simulink model "filter1"  (R2020b)
settings: Solver=VariableStepAuto  StartTime=0.0  StopTime=10.0  MaxStep=0.8  RelTol=1e-3
settings Model: Creator=Ravi  LastModifiedBy=Ravi
settings DataIOCC: SaveOutput=off  SaveTime=off

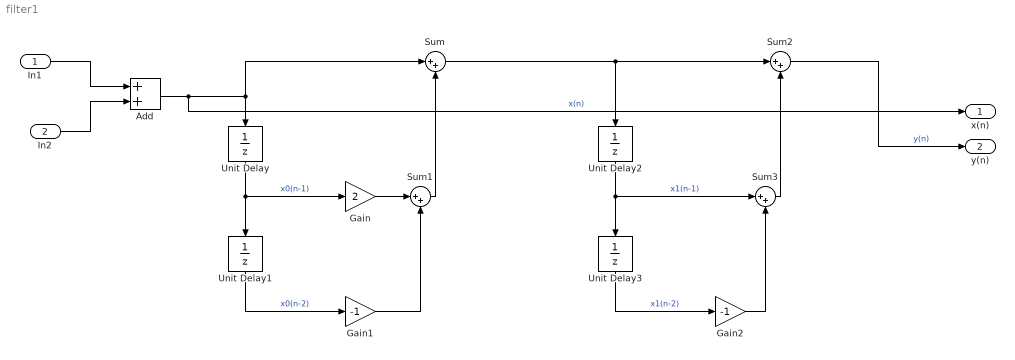
== system filter1 ==
  In1 : Inport  OutDataTypeStr=double  PortDimensions=1  SampleTime=0
  In2 : Inport  Port=2  OutDataTypeStr=double  PortDimensions=1  SampleTime=0
  Add : Sum
  Gain : Gain  Gain=2
  Gain1 : Gain  Gain=-1
  Gain2 : Gain  Gain=-1
  Sum{,1..3} (4 alike) : Sum  Inputs=|++
  Unit Delay{,1..3} (4 alike) : UnitDelay  SampleTime=-1  HasFrameUpgradeWarning=on
  x(n) : Outport  OutDataTypeStr=double  PortDimensions=1  SampleTime=0
  y(n) : Outport  Port=2  OutDataTypeStr=double  PortDimensions=1  SampleTime=0
  wires:
  Unit Delay/1 -> Unit Delay1/1, Gain/1  "x0(n-1)"
  Gain2/1 -> Sum3/2
  Unit Delay3/1 -> Gain2/1  "x1(n-2)"
  Unit Delay2/1 -> Unit Delay3/1, Sum3/1  "x1(n-1)"
  Sum1/1 -> Sum/2
  Add/1 -> Sum/1, Unit Delay/1, x(n)/1  "x(n)"
  Gain1/1 -> Sum1/2
  Unit Delay1/1 -> Gain1/1  "x0(n-2)"
  Sum3/1 -> Sum2/2
  Sum/1 -> Sum2/1, Unit Delay2/1
  In1/1 -> Add/1
  Gain/1 -> Sum1/1
  In2/1 -> Add/2
  Sum2/1 -> y(n)/1  "y(n)"
